simulink model "stateflow5"  (R2015a)
settings: Solver=ode45  StartTime=0.0  StopTime=10.0  RelTol=1e-3
values from neighbouring files (symbols this model uses):
  simout = [12 12 12 12 13 12 12 12 12 11 11 11 ... (97 elements, 97x1)]    [test_data_set2.mat]    (also in test_dataset_3.mat = [11 11 11 11 11 11 11 11 10 10 10 10 ... (67 elements, 67x1))
libraries: legoev3lib x2
settings Model: Creator=USER  LastModifiedBy=USER

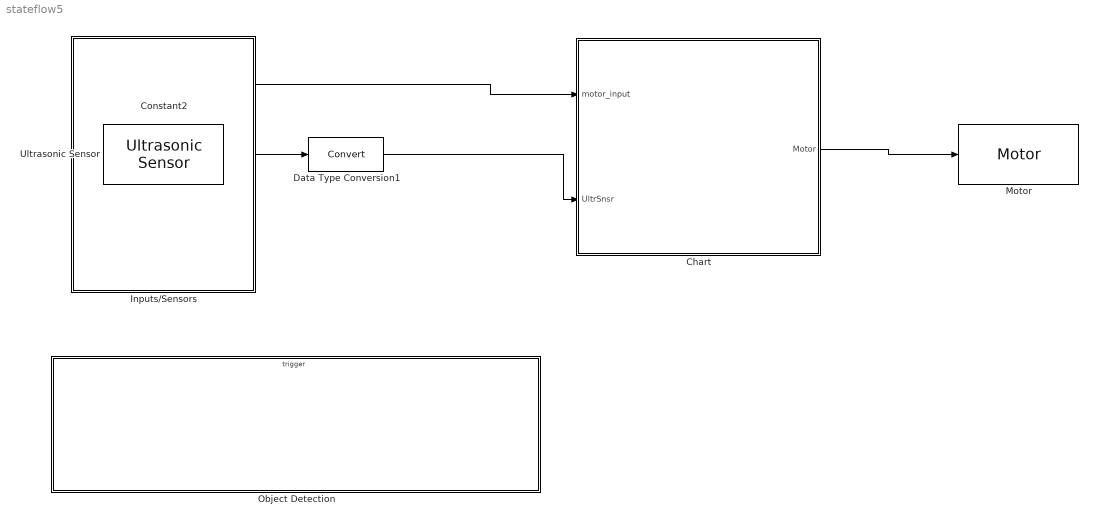
== system stateflow5 ==
  Chart : Stateflow chart  TreatAsAtomicUnit=on
  Constant2 : Constant  Value=20
  Data Type Conversion1 : DataTypeConversion
  Inputs/Sensors : Subsystem
  Motor : legoev3lib/Motor  sportNumber=A  sstopAction=Brake
  Object Detection : Subsystem  TreatAsAtomicUnit=on
  Ultrasonic Sensor : legoev3lib/Ultrasonic Sensor  PortNumber=1  sampleTime=0.01
  wires:
  Ultrasonic Sensor/1 -> Data Type Conversion1/1
  Data Type Conversion1/1 -> Chart/2(UltrSnsr)
  Constant2/1 -> Chart/1(motor_input)
  Chart/1(Motor) -> Motor/1

== system stateflow5/Inputs//Sensors ==

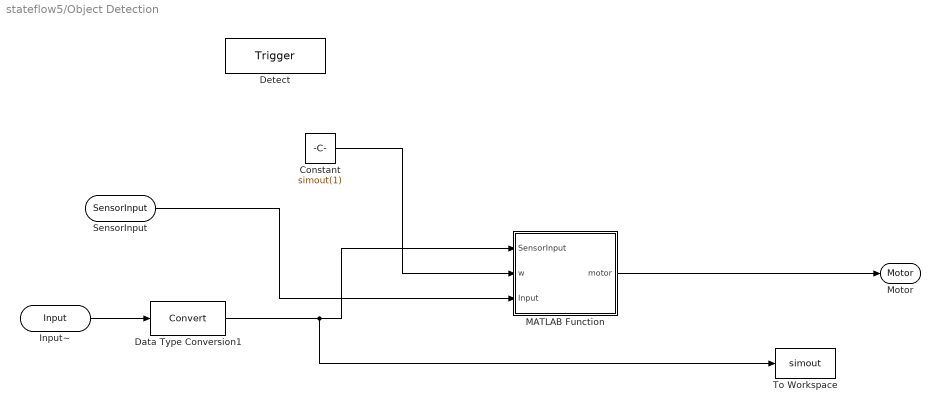
== system stateflow5/Object Detection ==
  Detect : TriggerPort  TriggerType=function-call  IsSimulinkFunction=on  FunctionName=Detect
  Constant : Constant  Value=simout(1)
  Data Type Conversion1 : DataTypeConversion
  MATLAB Function : MATLAB Function  TreatAsAtomicUnit=on
  To Workspace : ToWorkspace  VariableName=simout  SampleTime=-1
  Input~ : ArgIn  DisableCoverage=on  ArgumentName=Input
  SensorInput : ArgIn  DisableCoverage=on  Port=2  ArgumentName=SensorInput
  Motor : ArgOut  DisableCoverage=on  ArgumentName=Motor
  wires:
  MATLAB Function/1(motor) -> Motor/1
  Constant/1 -> MATLAB Function/2(w)
  SensorInput/1 -> MATLAB Function/3(Input)
  Input~/1 -> Data Type Conversion1/1
  Data Type Conversion1/1 -> To Workspace/1, MATLAB Function/1(SensorInput)

== matlab function stateflow5/Object Detection/MATLAB Function ==
  data: SensorInput input; motor output; w input; Input input
function motor = fcn(SensorInput,w,Input)
x=w;
if((SensorInput-x)>2)||((SensorInput-x)<-2)
    motor = 0;
else(SensorInput>4)&&(SensorInput<=20)
    motor = Input;
end
end

== stateflow chart stateflow5/Chart ==
  (default) -> (junction 19) : {Motor = Detect(motor_input,UltrSnsr)}
  (junction 19) -> (junction 29)
  data: motor_input input; Motor output; UltrSnsr input
